simulink model "July11thSecond"  (R2015a)
settings: Solver=ode45  StartTime=0.0  StopTime=10.0  RelTol=1e-3
PreLoadFcn:
  | SPParameters;
undefined symbols (not defined in the file or in its folder): Phiamp, Psiamp, Thetaamp, Xamp, Yamp, Zamp
settings Model: Creator=admin  LastModifiedBy=admin

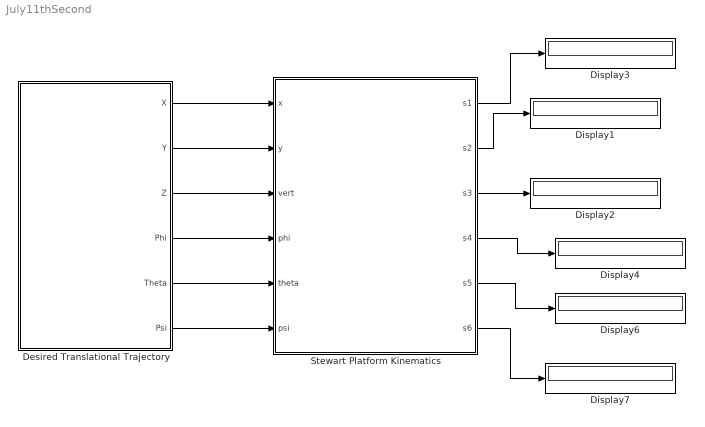
== system July11thSecond ==
  Desired Translational Trajectory : Subsystem
  Display{1..4,6..7} (6 alike) : Display
  Stewart Platform Kinematics : MATLAB Function  TreatAsAtomicUnit=on
  wires:
  Desired Translational Trajectory/1(X) -> Stewart Platform Kinematics/1(x)
  Desired Translational Trajectory/2(Y) -> Stewart Platform Kinematics/2(y)
  Desired Translational Trajectory/3(Z) -> Stewart Platform Kinematics/3(vert)
  Desired Translational Trajectory/4(Phi) -> Stewart Platform Kinematics/4(phi)
  Desired Translational Trajectory/5(Theta) -> Stewart Platform Kinematics/5(theta)
  Desired Translational Trajectory/6(Psi) -> Stewart Platform Kinematics/6(psi)
  Stewart Platform Kinematics/1(s1) -> Display3/1
  Stewart Platform Kinematics/2(s2) -> Display1/1
  Stewart Platform Kinematics/3(s3) -> Display2/1
  Stewart Platform Kinematics/4(s4) -> Display4/1
  Stewart Platform Kinematics/5(s5) -> Display6/1
  Stewart Platform Kinematics/6(s6) -> Display7/1

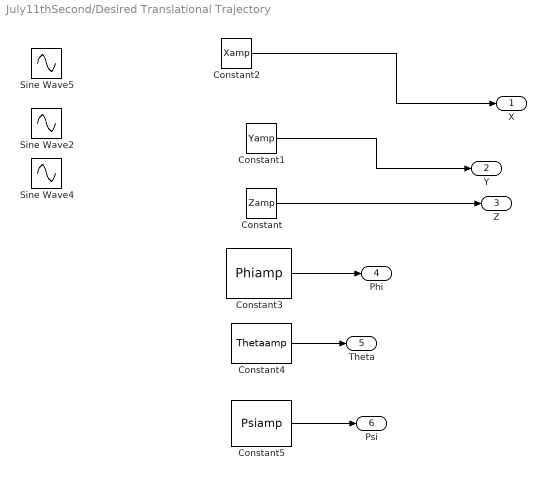
== system July11thSecond/Desired Translational Trajectory ==
  Constant : Constant  Value=Zamp
  Constant1 : Constant  Value=Yamp
  Constant2 : Constant  Value=Xamp
  Constant3 : Constant  Value=Phiamp
  Constant4 : Constant  Value=Thetaamp
  Constant5 : Constant  Value=Psiamp
  Sine Wave2 : Sin  Amplitude=Yamp  Frequency=5  SampleTime=0
  Sine Wave4 : Sin  Amplitude=Zamp  Frequency=5  SampleTime=0
  Sine Wave5 : Sin  Amplitude=Xamp  Frequency=5  SampleTime=0
  X : Outport
  Y : Outport  Port=2
  Z : Outport  Port=3
  Phi : Outport  Port=4
  Theta : Outport  Port=5
  Psi : Outport  Port=6
  wires:
  Constant/1 -> Z/1
  Constant2/1 -> X/1
  Constant1/1 -> Y/1
  Constant5/1 -> Psi/1
  Constant4/1 -> Theta/1
  Constant3/1 -> Phi/1

== matlab function July11thSecond/Stewart Platform Kinematics ==
  data: x input; y input; vert input; phi input; theta input; psi input; s1 output; s2 output; s3 output; s4 output; s5 output; s6 output
function [s1,s2,s3,s4,s5,s6] = fcn(x,y,vert,phi,theta,psi)

z=0.293+vert; %20cm is the distance between two platforms

%Define the system parameters

%gammap1 = 53.45 ; % unit in degree
gammap1=8;
gammap = [gammap1,120-gammap1, 120+gammap1, -120-gammap1,-120+gammap1,-gammap1];
gammab1 = 20; % unit in degree %onsidering servo arm length of 4.5cm
%gammab1 = 21.1495 ; % unit in degree
gammab = [gammab1,120-gammab1, 120+gammab1, -120-gammab1,-120+gammab1,-gammab1];
%beta=12.63*pi/180;
rp = 0.10; % radius of platform ,in meter
rb = 0.20;  % radius of base,in meter
hp = 0.01;   % platform nominal height ,in meter

s=0.045;   %Servo arm length in cm
len=0.3202;  %Leg length in cm
length=zeros(6,1);

spsi = sin(psi*pi/180 );
cpsi = cos(psi*pi/180 );
sthe = sin(theta*pi/180 );
cthe = cos(theta*pi/180 );
sphi = sin(phi*pi/180 );
cphi = cos(phi*pi/180 );
% rotation matrix R
bRp=zeros(3,3);
bRp(1,1 ) = cphi * cthe ;
bRp(1,2 ) = -sphi * cpsi + cphi * sthe * spsi ;
bRp(1,3 ) = sphi * spsi + cphi * sthe * cpsi ;
bRp(2,1 ) = sphi * cthe ;
bRp(2,2 ) = cphi * cpsi + sphi * sthe * spsi ;
bRp(2,3 ) = -cphi * spsi + sphi * sthe * cpsi ;
bRp(3,1 ) = -sthe ;
bRp(3,2 ) = cthe * spsi ;
bRp(3,3 ) = cthe * cpsi ;
% fixed vector of pp
bRp;
pp=zeros(3,6);
pp(1,: ) = rp*cos(gammap*pi/180);
pp(2,: ) = rp*sin(gammap*pi/180) ;
pp(3,: ) = [hp/2,hp/2,hp/2,hp/2,hp/2,hp/2 ] ;
pp;
%fixed vector of bb
bb=zeros(3,6);
bb(1,: ) = rb*cos(gammab*pi/180);
bb(2,: ) = rb*sin(gammab*pi/180) ;
bb(3,: ) = [0,0,0,0,0,0];
% bdp
bb;
bdp = [x,y,z ]' ;
bDp = [bdp,bdp,bdp,bdp,bdp,bdp] ;

bDp;
    
% actuator vector
qq=bRp*pp+bDp;
qq;
bA = bRp*pp +bDp - bb ;
bA;
L=zeros(3,6);
for i=1:6
   L(:,i)= rotationmat(gammab(1,i))*bA(:,i)-[rb,0,0]'; %Origin is shifted each time to the servo location
  rotationmat(gammab(1,i)) ;
end


for i =1:6 
length(i,1) = norm(bA(:,i)) ;
end
servoangt=zeros(6,2);
offset1=[10.2575,18.9046,10.2575,18.9046,10.2575,18.9046]';
offset2=[-180,-180,-180,-180,-180,-180]';
offset=[-8.1635,8.1635,-8.1635,8.1635,-8.1635,8.1635]';
for i=1:6
    a=2*s*L(2,i);
    b=2*s*L(3,i);
    c=len^2-(length(i,1))^2;
  
      
     servoangt(i,1)=(acos(-c/(sqrt(a^2+b^2)))+atan2(b,a))*180/pi+offset2(i,1)-10.2575;
 
    servoangt(i,2)=(-acos(-c/(sqrt(a^2+b^2)))+atan2(b,a))*(180/pi)+offset1(i,1);
end

servoang=zeros(6,1);
for i=1:6
    if(mod(i,2)==0)
        
    servoang(i,1)=servoangt(i,1)+offset(i,1);
    
    else
      servoang(i,1)=servoangt(i,2)+ offset(i,1);
    end
    
end



%[length,bA,servoang]=servoangles(x,y,z,psi,theta,phi);
s1=servoang(1,1);
s2=servoang(2,1);
s3=servoang(3,1);
s4=servoang(4,1);
s5=servoang(5,1);
s6=servoang(6,1);

bA;
length;

end

function[rot]=rotationmat(gamma)

rot=zeros(3,3);
rot(1,1)=cos(gamma*pi/180);
rot(1,2)=sin(gamma*pi/180);
rot(1,3)=0;
rot(2,1)=-sin(gamma*pi/180);
rot(2,2)=cos(gamma*pi/180);
rot(2,3)=0;
rot(3,1)=0;
rot(3,2)=0;
rot(3,3)=1;

end
